simulink model "problem4"  (R2022a)
settings: Solver=VariableStepAuto  StartTime=0.0  StopTime=4  RelTol=1e-3
libraries: simulink x2, simulink_extras x1
settings Model: Creator=Weilong Chen  LastModifiedBy=Weilong Chen

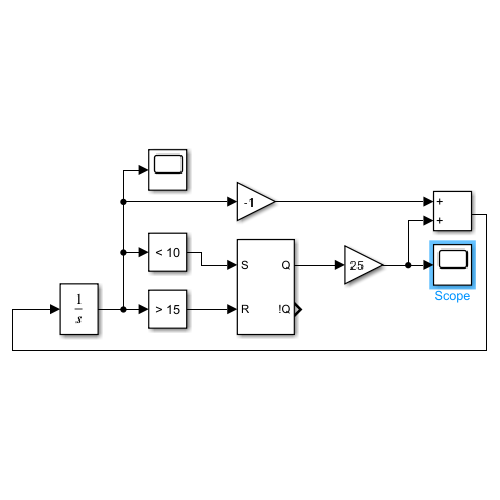
[thumbnail: Simulink's stored preview of the top-level diagram]
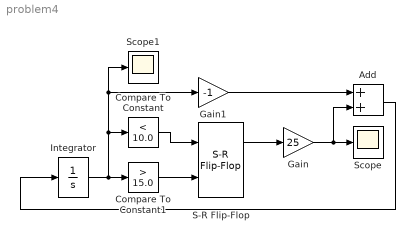
== system problem4 ==
  Add : Sum
  Compare To Constant : simulink/Logic and Bit Operations/Compare To Constant  relop=<  const=10.0  OutDataTypeStr=boolean
  Compare To Constant1 : simulink/Logic and Bit Operations/Compare To Constant  relop=>  const=15.0  OutDataTypeStr=boolean
  Gain : Gain  Gain=25
  Gain1 : Gain  Gain=-1
  Integrator : Integrator  InitialCondition=12
  S-R Flip-Flop : simulink_extras/Flip Flops/S-R Flip-Flop  initial_condition=0
  Scope : Scope
  Scope1 : Scope
  wires:
  S-R Flip-Flop/1 -> Gain/1
  Add/1 -> Integrator/1
  Gain1/1 -> Add/1
  Compare To Constant1/1 -> S-R Flip-Flop/2
  Gain/1 -> Add/2, Scope/1
  Compare To Constant/1 -> S-R Flip-Flop/1
  Integrator/1 -> Gain1/1, Scope1/1, Compare To Constant/1, Compare To Constant1/1
